simulink model "plantModel_th"  (R2020a)
settings: Solver=VariableStepAuto  StartTime=0.0  StopTime=0.25  MaxStep=0.05  RelTol=1e-3
values from neighbouring files (symbols this model uses):
  O_vWind = [20;0;0]    [plantModel_ts.m]
libraries: plantModel x1
settings Model: Creator=Ayaz  LastModifiedBy=Ayaz

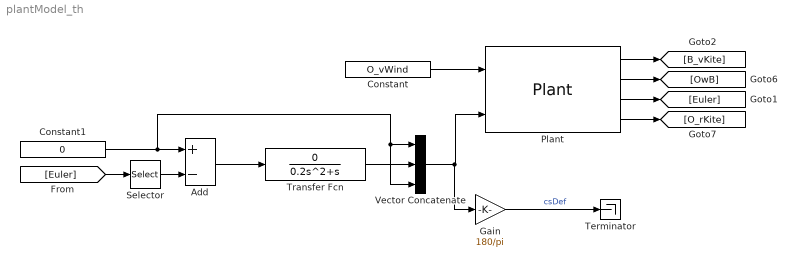
== system plantModel_th ==
  Add : Sum  Inputs=+-
  Constant : Constant  Value=O_vWind  VectorParams1D=off
  Constant1 : Constant  Value=0
  Gain : Gain  Gain=180/pi
  Plant : plantModel/Plant  mKite=mKite  jKite=jKite  refArea=refArea  refSpan=refSpan  refChord=refChord  gravAccl=gravAccl  rho=rho  init_rKite=init_O_rKite  init_B_vKite=init_B_vKite  init_Euler=init_Euler  init_OwB=init_OwB
      link override sixDoFDynamics: jKite=jKite  init_rKite=init_O_rKite  init_B_vKite=init_B_vKite  init_Euler=init_Euler  init_OwB=init_OwB
  Selector : Selector  InputPortWidth=3  IndexOptions=Index vector (dialog)  Indices=2  OutputSizes=1
  Terminator : Terminator
  Transfer Fcn : TransferFcn  Numerator=[0 0 -0]  Denominator=[0.2 1 0]
  Vector Concatenate : Concatenate  NumInputs=3
  wires:
  Constant/1 -> Plant/1
  Plant/2 -> [OwB]
  Plant/1 -> [B_vKite]
  Plant/3 -> [Euler]
  Plant/4 -> [O_rKite]
  [Euler] -> Selector/1
  Selector/1 -> Add/2
  Constant1/1 -> Vector Concatenate/3, Vector Concatenate/1, Add/1
  Add/1 -> Transfer Fcn/1
  Transfer Fcn/1 -> Vector Concatenate/2
  Vector Concatenate/1 -> Gain/1, Plant/2
  Gain/1 -> Terminator/1  "csDef"
